simulink model "AutoTuneOP"  (Simulink 7.0)
settings: Solver=ode3  StartTime=0.0  StopTime=2500  FixedStep=0.2  RelTol=1e-3
undefined symbols (not defined in the file or in its folder): buttonSim, disturbanceSim, relayBut, setSimA, tuningfunc3
settings Model: Creator=ismt  LastModifiedBy=ismt
settings DataIOCC: LimitDataPoints=off

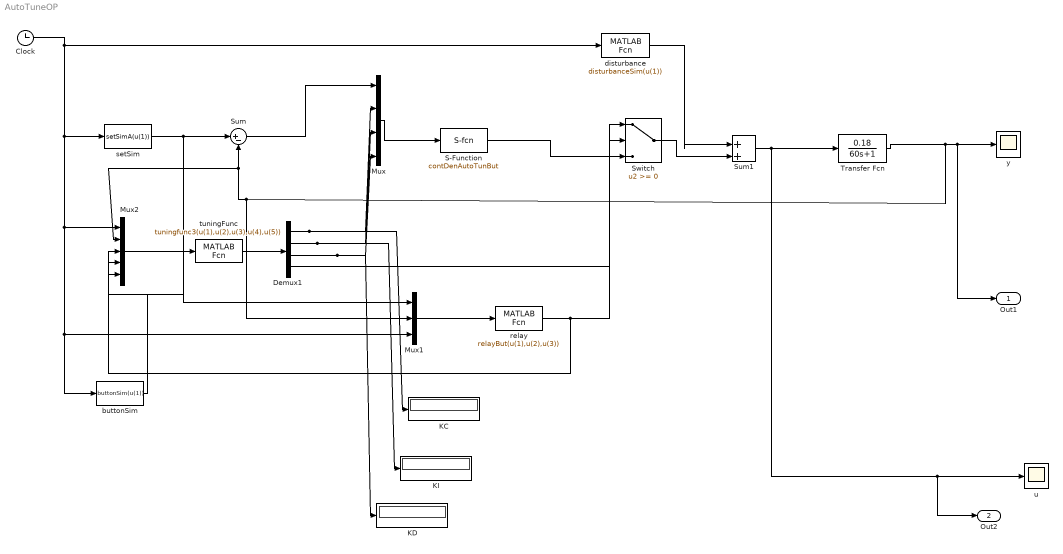
== system AutoTuneOP ==
  Clock : Clock
      settings: Decimation=10
  Demux1 : Demux
  KC : Display
  KD : Display
  KI : Display
  Mux : Mux
  Mux1 : Mux  Inputs=3
  Mux2 : Mux  Inputs=5
  S-Function : S-Function  FunctionName=contDenAutoTunBut
  Sum : Sum  Inputs=|+-  OutDataType=sfix(16)  OutScaling=2^0
  Sum1 : Sum  Inputs=|++  OutDataType=sfix(16)  OutScaling=2^0
  Switch : Switch  OutDataType=sfix(16)  OutScaling=2^0  SampleTime=0.2
  Transfer Fcn : TransferFcn  Numerator=[0.18]  Denominator=[60 1]
  buttonSim : MATLABFcn  MATLABFcn=buttonSim(u(1))  SampleTime=0.2
  disturbance : MATLABFcn  MATLABFcn=disturbanceSim(u(1))  SampleTime=0.2
  relay : MATLABFcn  MATLABFcn=relayBut(u(1),u(2),u(3))  SampleTime=0.2
  setSim : MATLABFcn  MATLABFcn=setSimA(u(1))  SampleTime=0.2
  tuningFunc : MATLABFcn  MATLABFcn=tuningfunc3(u(1),u(2),u(3),u(4),u(5))  SampleTime=0.2
  u : Scope
  y : Scope
  Out1 : Outport  OutDataType=sfix(16)  OutScaling=2^0
  Out2 : Outport  Port=2  OutDataType=sfix(16)  OutScaling=2^0
  wires:
  Sum1/1 -> Transfer Fcn/1, u/1, Out2/1
  S-Function/1 -> Switch/3
  relay/1 -> Switch/1, Mux2/5
  Clock/1 -> setSim/1, Mux2/1, buttonSim/1, Mux1/3, disturbance/1
  setSim/1 -> Sum/1, Mux2/4, Mux1/1
  Mux1/1 -> relay/1
  Transfer Fcn/1 -> Sum/2, Mux2/2, Mux1/2, y/1, Out1/1
  Sum/1 -> Mux/1
  Mux/1 -> S-Function/1
  buttonSim/1 -> Mux2/3
  Mux2/1 -> tuningFunc/1
  tuningFunc/1 -> Demux1/1
  Demux1/1 -> KC/1, Mux/2
  Demux1/2 -> Mux/3, KI/1
  Demux1/3 -> Mux/4, KD/1
  Demux1/4 -> Switch/2
  Switch/1 -> Sum1/2
  disturbance/1 -> Sum1/1
